simulink model "lab_02"  (R2020b)
settings: Solver=VariableStepAuto  StartTime=0.0  StopTime=10  RelTol=1e-3
libraries: simulink x1
settings Model: Creator=pawel  LastModifiedBy=pawel

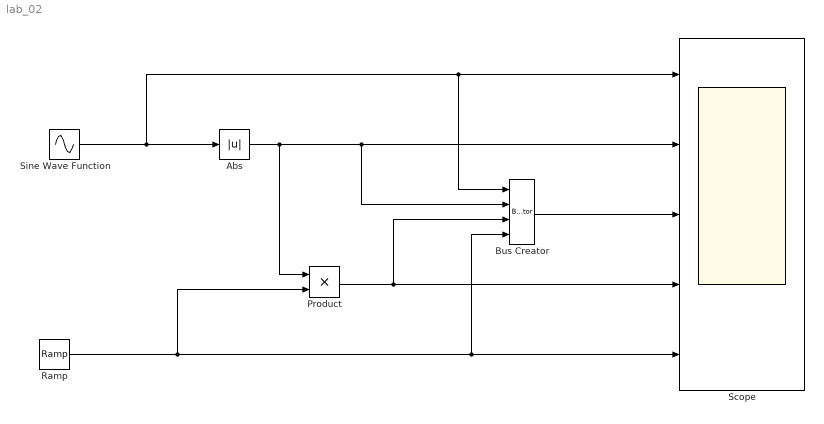
== system lab_02 ==
  Abs : Abs
  Bus Creator : BusCreator  Inputs=4
  Product : Product
  Ramp : simulink/Sources/Ramp  slope=1  start=0  InitialOutput=-1
  Scope : Scope  NumInputPorts=5
  Sine Wave Function : Sin  Frequency=2*2*pi  SampleTime=0
  wires:
  Sine Wave Function/1 -> Bus Creator/1, Scope/1, Abs/1
  Abs/1 -> Bus Creator/2, Scope/2, Product/1
  Ramp/1 -> Bus Creator/4, Scope/5, Product/2
  Product/1 -> Bus Creator/3, Scope/4
  Bus Creator/1 -> Scope/3
